simulink model "PV_string_with_MPPT"  (Simulink 8.8)
settings: Solver=ode3  StartTime=0.0  StopTime=600  FixedStep=1e-2  MaxStep=1e-4  RelTol=1e-5  EnableMultiTasking=on
(part 1 of 2)
settings Model: Creator=amaki  LastModifiedBy=jarvela7
settings DataIOCC: LimitDataPoints=off  SaveOutput=off  SaveTime=off
settings OptimizationCC: BooleanDataType=off  ExpressionDepthLimit=2147483647
settings DebuggingCC: AlgebraicLoopMsg=none
settings ConfigComp: CovSFcnEnable=off

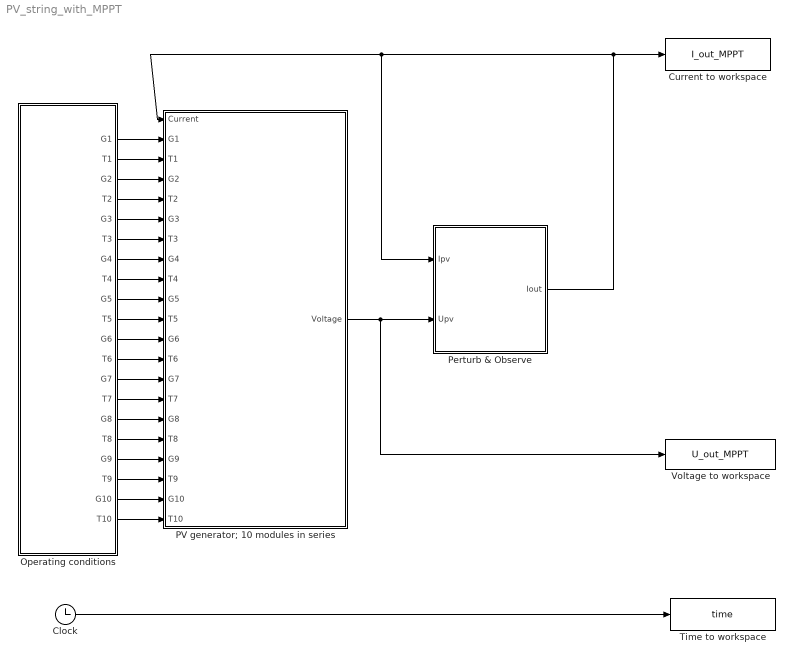
== system PV_string_with_MPPT ==
  Clock : Clock
  Current to workspace : ToWorkspace  VariableName=I_out_MPPT  SampleTime=-1
  Operating conditions : Subsystem
  PV generator; 10 modules in series : Subsystem
  Perturb & Observe : Subsystem  mask{pert_freq=1, pert_size=0.05}
      mask prompts: pert_freq "Perturbation frequency (Hz)"; pert_size "Perturbation step size (A)"
  Time to workspace : ToWorkspace  VariableName=time  SampleTime=-1
  Voltage to workspace : ToWorkspace  VariableName=U_out_MPPT  SampleTime=-1
  wires:
  Operating conditions/1(G1) -> PV generator; 10 modules in series/2(G1)
  Operating conditions/2(T1) -> PV generator; 10 modules in series/3(T1)
  Operating conditions/3(G2) -> PV generator; 10 modules in series/4(G2)
  Operating conditions/4(T2) -> PV generator; 10 modules in series/5(T2)
  Operating conditions/5(G3) -> PV generator; 10 modules in series/6(G3)
  Operating conditions/6(T3) -> PV generator; 10 modules in series/7(T3)
  Operating conditions/7(G4) -> PV generator; 10 modules in series/8(G4)
  Operating conditions/8(T4) -> PV generator; 10 modules in series/9(T4)
  Operating conditions/9(G5) -> PV generator; 10 modules in series/10(G5)
  Operating conditions/10(T5) -> PV generator; 10 modules in series/11(T5)
  Operating conditions/11(G6) -> PV generator; 10 modules in series/12(G6)
  Operating conditions/12(T6) -> PV generator; 10 modules in series/13(T6)
  Operating conditions/13(G7) -> PV generator; 10 modules in series/14(G7)
  Operating conditions/14(T7) -> PV generator; 10 modules in series/15(T7)
  Operating conditions/15(G8) -> PV generator; 10 modules in series/16(G8)
  Operating conditions/16(T8) -> PV generator; 10 modules in series/17(T8)
  Operating conditions/17(G9) -> PV generator; 10 modules in series/18(G9)
  Operating conditions/18(T9) -> PV generator; 10 modules in series/19(T9)
  Operating conditions/19(G10) -> PV generator; 10 modules in series/20(G10)
  Operating conditions/20(T10) -> PV generator; 10 modules in series/21(T10)
  Clock/1 -> Time to workspace/1
  PV generator; 10 modules in series/1(Voltage) -> Voltage to workspace/1, Perturb & Observe/2(Upv)
  Perturb & Observe/1(Iout) -> Current to workspace/1, PV generator; 10 modules in series/1(Current), Perturb & Observe/1(Ipv)

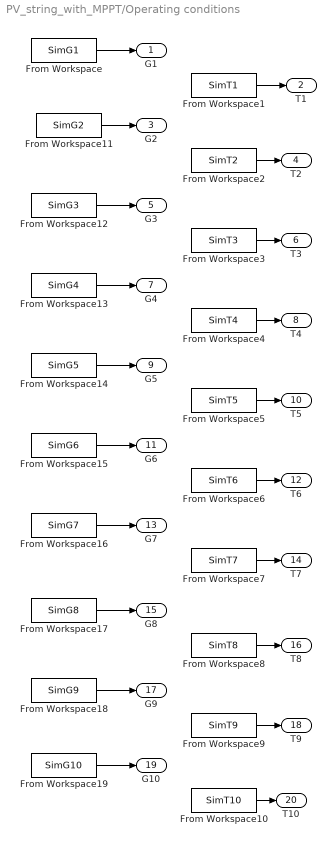
== system PV_string_with_MPPT/Operating conditions ==
  From Workspace : FromWorkspace  VariableName=SimG1  SampleTime=0
  From Workspace1 : FromWorkspace  VariableName=SimT1  SampleTime=0
  From Workspace10 : FromWorkspace  VariableName=SimT10  SampleTime=0
  From Workspace11 : FromWorkspace  VariableName=SimG2  SampleTime=0
  From Workspace12 : FromWorkspace  VariableName=SimG3  SampleTime=0
  From Workspace13 : FromWorkspace  VariableName=SimG4  SampleTime=0
  From Workspace14 : FromWorkspace  VariableName=SimG5  SampleTime=0
  From Workspace15 : FromWorkspace  VariableName=SimG6  SampleTime=0
  From Workspace16 : FromWorkspace  VariableName=SimG7  SampleTime=0
  From Workspace17 : FromWorkspace  VariableName=SimG8  SampleTime=0
  From Workspace18 : FromWorkspace  VariableName=SimG9  SampleTime=0
  From Workspace19 : FromWorkspace  VariableName=SimG10  SampleTime=0
  From Workspace2 : FromWorkspace  VariableName=SimT2  SampleTime=0
  From Workspace3 : FromWorkspace  VariableName=SimT3  SampleTime=0
  From Workspace4 : FromWorkspace  VariableName=SimT4  SampleTime=0
  From Workspace5 : FromWorkspace  VariableName=SimT5  SampleTime=0
  From Workspace6 : FromWorkspace  VariableName=SimT6  SampleTime=0
  From Workspace7 : FromWorkspace  VariableName=SimT7  SampleTime=0
  From Workspace8 : FromWorkspace  VariableName=SimT8  SampleTime=0
  From Workspace9 : FromWorkspace  VariableName=SimT9  SampleTime=0
  G1 : Outport
  T1 : Outport  Port=2
  G2 : Outport  Port=3
  T2 : Outport  Port=4
  G3 : Outport  Port=5
  T3 : Outport  Port=6
  G4 : Outport  Port=7
  T4 : Outport  Port=8
  G5 : Outport  Port=9
  T5 : Outport  Port=10
  G6 : Outport  Port=11
  T6 : Outport  Port=12
  G7 : Outport  Port=13
  T7 : Outport  Port=14
  G8 : Outport  Port=15
  T8 : Outport  Port=16
  G9 : Outport  Port=17
  T9 : Outport  Port=18
  G10 : Outport  Port=19
  T10 : Outport  Port=20
  wires:
  From Workspace1/1 -> T1/1
  From Workspace2/1 -> T2/1
  From Workspace3/1 -> T3/1
  From Workspace4/1 -> T4/1
  From Workspace5/1 -> T5/1
  From Workspace15/1 -> G6/1
  From Workspace6/1 -> T6/1
  From Workspace16/1 -> G7/1
  From Workspace7/1 -> T7/1
  From Workspace17/1 -> G8/1
  From Workspace8/1 -> T8/1
  From Workspace18/1 -> G9/1
  From Workspace9/1 -> T9/1
  From Workspace10/1 -> T10/1
  From Workspace19/1 -> G10/1
  From Workspace/1 -> G1/1
  From Workspace11/1 -> G2/1
  From Workspace12/1 -> G3/1
  From Workspace13/1 -> G4/1
  From Workspace14/1 -> G5/1

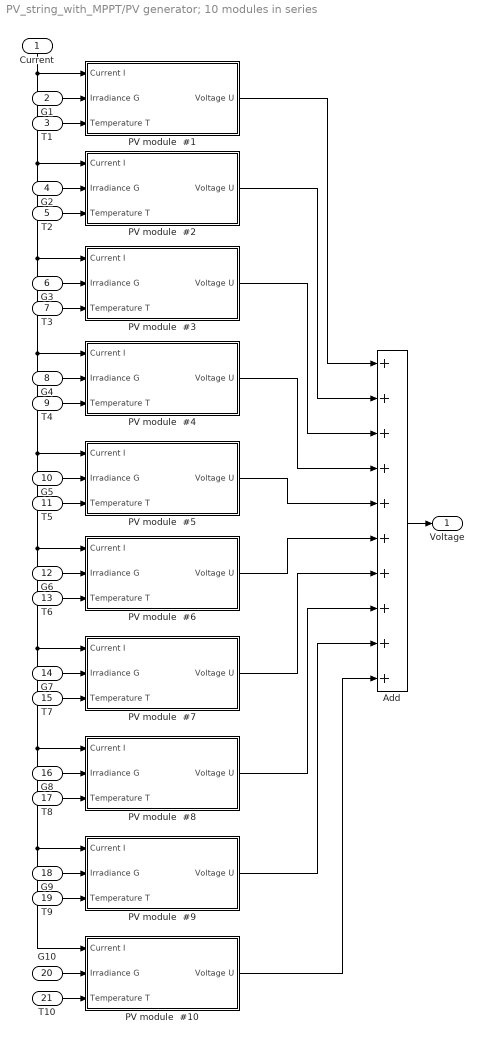
== system PV_string_with_MPPT/PV generator; 10 modules in series ==
  Current : Inport
  G1 : Inport  Port=2
  T1 : Inport  Port=3
  G2 : Inport  Port=4
  T2 : Inport  Port=5
  G3 : Inport  Port=6
  T3 : Inport  Port=7
  G4 : Inport  Port=8
  T4 : Inport  Port=9
  G5 : Inport  Port=10
  T5 : Inport  Port=11
  G6 : Inport  Port=12
  T6 : Inport  Port=13
  G7 : Inport  Port=14
  T7 : Inport  Port=15
  G8 : Inport  Port=16
  T8 : Inport  Port=17
  G9 : Inport  Port=18
  T9 : Inport  Port=19
  G10 : Inport  Port=20
  T10 : Inport  Port=21
  Add : Sum  Inputs=++++++++++
  PV module  #1 : Subsystem  mask{Isc_stc=8.02, Uoc_stc=33.1, G_stc=1000, T_stc=273.15+25, Ns=54, Rs=0.329385084266289, Rsh=187.8287416854189, A=1.3, Ku=-0.1242, Ki=0.0047, k=1.3806503e-23, q=1.60217646e-19}
      mask prompts: Isc_stc "STC short-circuit current"; Uoc_stc "STC open-circuit voltage"; G_stc "STC irradiance"; T_stc "STC temperature"; Ns "Number of cells"; Rs "Series resistance Rs"; Rsh "Shunt resistance Rsh"; A "Ideality factor A"; Ku "Temp. coeff. of OC Ku"; Ki "Temp. coeff. of SC Ki"; k "Boltzmann constant"; q "Elementary charge"
  PV module  #10 : Subsystem  mask{Isc_stc=8.02, Uoc_stc=33.1, G_stc=1000, T_stc=273.15+25, Ns=54, Rs=0.329385084266289, Rsh=187.8287416854189, A=1.3, Ku=-0.1242, Ki=0.0047, k=1.3806503e-23, q=1.60217646e-19}
      mask prompts: Isc_stc "STC short-circuit current"; Uoc_stc "STC open-circuit voltage"; G_stc "STC irradiance"; T_stc "STC temperature"; Ns "Number of cells"; Rs "Series resistance Rs"; Rsh "Shunt resistance Rsh"; A "Ideality factor A"; Ku "Temp. coeff. of OC Ku"; Ki "Temp. coeff. of SC Ki"; k "Boltzmann constant"; q "Elementary charge"
  PV module  #2 : Subsystem  mask{Isc_stc=8.02, Uoc_stc=33.1, G_stc=1000, T_stc=273.15+25, Ns=54, Rs=0.329385084266289, Rsh=187.8287416854189, A=1.3, Ku=-0.1242, Ki=0.0047, k=1.3806503e-23, q=1.60217646e-19}
      mask prompts: Isc_stc "STC short-circuit current"; Uoc_stc "STC open-circuit voltage"; G_stc "STC irradiance"; T_stc "STC temperature"; Ns "Number of cells"; Rs "Series resistance Rs"; Rsh "Shunt resistance Rsh"; A "Ideality factor A"; Ku "Temp. coeff. of OC Ku"; Ki "Temp. coeff. of SC Ki"; k "Boltzmann constant"; q "Elementary charge"
  PV module  #3 : Subsystem  mask{Isc_stc=8.02, Uoc_stc=33.1, G_stc=1000, T_stc=273.15+25, Ns=54, Rs=0.329385084266289, Rsh=187.8287416854189, A=1.3, Ku=-0.1242, Ki=0.0047, k=1.3806503e-23, q=1.60217646e-19}
      mask prompts: Isc_stc "STC short-circuit current"; Uoc_stc "STC open-circuit voltage"; G_stc "STC irradiance"; T_stc "STC temperature"; Ns "Number of cells"; Rs "Series resistance Rs"; Rsh "Shunt resistance Rsh"; A "Ideality factor A"; Ku "Temp. coeff. of OC Ku"; Ki "Temp. coeff. of SC Ki"; k "Boltzmann constant"; q "Elementary charge"
  PV module  #4 : Subsystem  mask{Isc_stc=8.02, Uoc_stc=33.1, G_stc=1000, T_stc=273.15+25, Ns=54, Rs=0.329385084266289, Rsh=187.8287416854189, A=1.3, Ku=-0.1242, Ki=0.0047, k=1.3806503e-23, q=1.60217646e-19}
      mask prompts: Isc_stc "STC short-circuit current"; Uoc_stc "STC open-circuit voltage"; G_stc "STC irradiance"; T_stc "STC temperature"; Ns "Number of cells"; Rs "Series resistance Rs"; Rsh "Shunt resistance Rsh"; A "Ideality factor A"; Ku "Temp. coeff. of OC Ku"; Ki "Temp. coeff. of SC Ki"; k "Boltzmann constant"; q "Elementary charge"
  PV module  #5 : Subsystem  mask{Isc_stc=8.02, Uoc_stc=33.1, G_stc=1000, T_stc=273.15+25, Ns=54, Rs=0.329385084266289, Rsh=187.8287416854189, A=1.3, Ku=-0.1242, Ki=0.0047, k=1.3806503e-23, q=1.60217646e-19}
      mask prompts: Isc_stc "STC short-circuit current"; Uoc_stc "STC open-circuit voltage"; G_stc "STC irradiance"; T_stc "STC temperature"; Ns "Number of cells"; Rs "Series resistance Rs"; Rsh "Shunt resistance Rsh"; A "Ideality factor A"; Ku "Temp. coeff. of OC Ku"; Ki "Temp. coeff. of SC Ki"; k "Boltzmann constant"; q "Elementary charge"
  PV module  #6 : Subsystem  mask{Isc_stc=8.02, Uoc_stc=33.1, G_stc=1000, T_stc=273.15+25, Ns=54, Rs=0.329385084266289, Rsh=187.8287416854189, A=1.3, Ku=-0.1242, Ki=0.0047, k=1.3806503e-23, q=1.60217646e-19}
      mask prompts: Isc_stc "STC short-circuit current"; Uoc_stc "STC open-circuit voltage"; G_stc "STC irradiance"; T_stc "STC temperature"; Ns "Number of cells"; Rs "Series resistance Rs"; Rsh "Shunt resistance Rsh"; A "Ideality factor A"; Ku "Temp. coeff. of OC Ku"; Ki "Temp. coeff. of SC Ki"; k "Boltzmann constant"; q "Elementary charge"
  PV module  #7 : Subsystem  mask{Isc_stc=8.02, Uoc_stc=33.1, G_stc=1000, T_stc=273.15+25, Ns=54, Rs=0.329385084266289, Rsh=187.8287416854189, A=1.3, Ku=-0.1242, Ki=0.0047, k=1.3806503e-23, q=1.60217646e-19}
      mask prompts: Isc_stc "STC short-circuit current"; Uoc_stc "STC open-circuit voltage"; G_stc "STC irradiance"; T_stc "STC temperature"; Ns "Number of cells"; Rs "Series resistance Rs"; Rsh "Shunt resistance Rsh"; A "Ideality factor A"; Ku "Temp. coeff. of OC Ku"; Ki "Temp. coeff. of SC Ki"; k "Boltzmann constant"; q "Elementary charge"
  PV module  #8 : Subsystem  mask{Isc_stc=8.02, Uoc_stc=33.1, G_stc=1000, T_stc=273.15+25, Ns=54, Rs=0.329385084266289, Rsh=187.8287416854189, A=1.3, Ku=-0.1242, Ki=0.0047, k=1.3806503e-23, q=1.60217646e-19}
      mask prompts: Isc_stc "STC short-circuit current"; Uoc_stc "STC open-circuit voltage"; G_stc "STC irradiance"; T_stc "STC temperature"; Ns "Number of cells"; Rs "Series resistance Rs"; Rsh "Shunt resistance Rsh"; A "Ideality factor A"; Ku "Temp. coeff. of OC Ku"; Ki "Temp. coeff. of SC Ki"; k "Boltzmann constant"; q "Elementary charge"
  PV module  #9 : Subsystem  mask{Isc_stc=8.02, Uoc_stc=33.1, G_stc=1000, T_stc=273.15+25, Ns=54, Rs=0.329385084266289, Rsh=187.8287416854189, A=1.3, Ku=-0.1242, Ki=0.0047, k=1.3806503e-23, q=1.60217646e-19}
      mask prompts: Isc_stc "STC short-circuit current"; Uoc_stc "STC open-circuit voltage"; G_stc "STC irradiance"; T_stc "STC temperature"; Ns "Number of cells"; Rs "Series resistance Rs"; Rsh "Shunt resistance Rsh"; A "Ideality factor A"; Ku "Temp. coeff. of OC Ku"; Ki "Temp. coeff. of SC Ki"; k "Boltzmann constant"; q "Elementary charge"
  Voltage : Outport
  wires:
  PV module  #1/1(Voltage U) -> Add/1
  PV module  #2/1(Voltage U) -> Add/2
  PV module  #3/1(Voltage U) -> Add/3
  PV module  #4/1(Voltage U) -> Add/4
  PV module  #5/1(Voltage U) -> Add/5
  PV module  #6/1(Voltage U) -> Add/6
  PV module  #7/1(Voltage U) -> Add/7
  PV module  #8/1(Voltage U) -> Add/8
  PV module  #9/1(Voltage U) -> Add/9
  PV module  #10/1(Voltage U) -> Add/10
  Current/1 -> PV module  #1/1(Current I), PV module  #2/1(Current I), PV module  #3/1(Current I), PV module  #4/1(Current I), PV module  #5/1(Current I), PV module  #6/1(Current I), PV module  #7/1(Current I), PV module  #8/1(Current I), PV module  #9/1(Current I), PV module  #10/1(Current I)
  G1/1 -> PV module  #1/2(Irradiance G)
  T1/1 -> PV module  #1/3(Temperature T)
  G2/1 -> PV module  #2/2(Irradiance G)
  T2/1 -> PV module  #2/3(Temperature T)
  G3/1 -> PV module  #3/2(Irradiance G)
  T3/1 -> PV module  #3/3(Temperature T)
  G4/1 -> PV module  #4/2(Irradiance G)
  T4/1 -> PV module  #4/3(Temperature T)
  G5/1 -> PV module  #5/2(Irradiance G)
  T5/1 -> PV module  #5/3(Temperature T)
  Add/1 -> Voltage/1
  G6/1 -> PV module  #6/2(Irradiance G)
  T6/1 -> PV module  #6/3(Temperature T)
  G7/1 -> PV module  #7/2(Irradiance G)
  T7/1 -> PV module  #7/3(Temperature T)
  G8/1 -> PV module  #8/2(Irradiance G)
  T8/1 -> PV module  #8/3(Temperature T)
  G9/1 -> PV module  #9/2(Irradiance G)
  T9/1 -> PV module  #9/3(Temperature T)
  G10/1 -> PV module  #10/2(Irradiance G)
  T10/1 -> PV module  #10/3(Temperature T)

== system PV_string_with_MPPT/Perturb & Observe ==
  Ipv : Inport
  Upv : Inport  Port=2
  Memory : Memory  InheritSampleTime=on
  Memory1 : Memory  InheritSampleTime=on
  Memory3 : Memory  X0=0.1  InheritSampleTime=on
  P : Product  RndMeth=Zero
  Product : Product  RndMeth=Zero
  Product1 : Product  RndMeth=Zero
  Rate Transition : RateTransition  OutPortSampleTime=1e-2
  Saturation : Saturate  UpperLimit=inf  LowerLimit=0
  Sign : Signum
  Sign1 : Signum
  Sign2 : Signum
  Sum : Sum  Inputs=|++
  Zero-Order Hold : ZeroOrderHold  SampleTime=1/pert_freq
  Zero-Order Hold1 : ZeroOrderHold  SampleTime=1/pert_freq
  dp : Sum  Inputs=+-
  du : Sum  Inputs=+-
  step : Constant  Value=-pert_size
  Iout : Outport
  wires:
  Memory1/1 -> du/2
  Memory/1 -> dp/2
  Upv/1 -> Zero-Order Hold1/1
  du/1 -> Sign1/1
  step/1 -> Product/2
  Product/1 -> Sum/1
  Sign/1 -> Product1/1
  Sign1/1 -> Product1/2
  Product1/1 -> Sign2/1
  Ipv/1 -> Zero-Order Hold/1
  Zero-Order Hold1/1 -> P/2, Memory1/1, du/1
  Zero-Order Hold/1 -> P/1
  P/1 -> Memory/1, dp/1
  dp/1 -> Sign/1
  Sign2/1 -> Product/1
  Sum/1 -> Rate Transition/1, Memory3/1
  Rate Transition/1 -> Saturation/1
  Memory3/1 -> Sum/2
  Saturation/1 -> Iout/1

== system PV_string_with_MPPT/PV generator; 10 modules in series/PV module  #1 ==
  Current I : Inport
  Irradiance G : Inport  Port=2
  Temperature T : Inport  Port=3
  Add1 : Sum  Inputs=-+
  Bypass diode : Subsystem  mask{k=1.3806503e-23, q=1.60217646e-19, Rs_bypass=0.02}
      mask prompts: k "Boltzmann constant"; q "Elementary charge"; Rs_bypass "Series resistance"
  MinMax : MinMax  Function=max  Inputs=2
  Pv module : Subsystem
  Voltage U : Outport
  wires:
  MinMax/1 -> Voltage U/1
  Add1/1 -> Bypass diode/1(I)
  Bypass diode/1(Ubypass) -> MinMax/2
  Pv module/2(Isc) -> Add1/1
  Pv module/1(U) -> MinMax/1
  Irradiance G/1 -> Pv module/1(G)
  Temperature T/1 -> Pv module/2(T)
  Current I/1 -> Pv module/3(I), Add1/2

== system PV_string_with_MPPT/PV generator; 10 modules in series/PV module  #10 ==
  Current I : Inport
  Irradiance G : Inport  Port=2
  Temperature T : Inport  Port=3
  Add1 : Sum  Inputs=-+
  Bypass diode : Subsystem  mask{k=1.3806503e-23, q=1.60217646e-19, Rs_bypass=0.02}
      mask prompts: k "Boltzmann constant"; q "Elementary charge"; Rs_bypass "Series resistance"
  MinMax : MinMax  Function=max  Inputs=2
  Pv module : Subsystem
  Voltage U : Outport
  wires:
  MinMax/1 -> Voltage U/1
  Add1/1 -> Bypass diode/1(I)
  Bypass diode/1(Ubypass) -> MinMax/2
  Pv module/2(Isc) -> Add1/1
  Pv module/1(U) -> MinMax/1
  Irradiance G/1 -> Pv module/1(G)
  Temperature T/1 -> Pv module/2(T)
  Current I/1 -> Pv module/3(I), Add1/2

== system PV_string_with_MPPT/PV generator; 10 modules in series/PV module  #2 ==
  Current I : Inport
  Irradiance G : Inport  Port=2
  Temperature T : Inport  Port=3
  Add1 : Sum  Inputs=-+
  Bypass diode : Subsystem  mask{k=1.3806503e-23, q=1.60217646e-19, Rs_bypass=0.02}
      mask prompts: k "Boltzmann constant"; q "Elementary charge"; Rs_bypass "Series resistance"
  MinMax : MinMax  Function=max  Inputs=2
  Pv module : Subsystem
  Voltage U : Outport
  wires:
  Current I/1 -> Add1/2, Pv module/3(I)
  Temperature T/1 -> Pv module/2(T)
  Irradiance G/1 -> Pv module/1(G)
  Pv module/1(U) -> MinMax/1
  Pv module/2(Isc) -> Add1/1
  Bypass diode/1(Ubypass) -> MinMax/2
  Add1/1 -> Bypass diode/1(I)
  MinMax/1 -> Voltage U/1

== system PV_string_with_MPPT/PV generator; 10 modules in series/PV module  #3 ==
  Current I : Inport
  Irradiance G : Inport  Port=2
  Temperature T : Inport  Port=3
  Add1 : Sum  Inputs=-+
  Bypass diode : Subsystem  mask{k=1.3806503e-23, q=1.60217646e-19, Rs_bypass=0.02}
      mask prompts: k "Boltzmann constant"; q "Elementary charge"; Rs_bypass "Series resistance"
  MinMax : MinMax  Function=max  Inputs=2
  Pv module : Subsystem
  Voltage U : Outport
  wires:
  MinMax/1 -> Voltage U/1
  Add1/1 -> Bypass diode/1(I)
  Bypass diode/1(Ubypass) -> MinMax/2
  Pv module/2(Isc) -> Add1/1
  Pv module/1(U) -> MinMax/1
  Irradiance G/1 -> Pv module/1(G)
  Temperature T/1 -> Pv module/2(T)
  Current I/1 -> Pv module/3(I), Add1/2

== system PV_string_with_MPPT/PV generator; 10 modules in series/PV module  #4 ==
  Current I : Inport
  Irradiance G : Inport  Port=2
  Temperature T : Inport  Port=3
  Add1 : Sum  Inputs=-+
  Bypass diode : Subsystem  mask{k=1.3806503e-23, q=1.60217646e-19, Rs_bypass=0.02}
      mask prompts: k "Boltzmann constant"; q "Elementary charge"; Rs_bypass "Series resistance"
  MinMax : MinMax  Function=max  Inputs=2
  Pv module : Subsystem
  Voltage U : Outport
  wires:
  Current I/1 -> Add1/2, Pv module/3(I)
  Temperature T/1 -> Pv module/2(T)
  Irradiance G/1 -> Pv module/1(G)
  Pv module/1(U) -> MinMax/1
  Pv module/2(Isc) -> Add1/1
  Bypass diode/1(Ubypass) -> MinMax/2
  Add1/1 -> Bypass diode/1(I)
  MinMax/1 -> Voltage U/1

== system PV_string_with_MPPT/PV generator; 10 modules in series/PV module  #5 ==
  Current I : Inport
  Irradiance G : Inport  Port=2
  Temperature T : Inport  Port=3
  Add1 : Sum  Inputs=-+
  Bypass diode : Subsystem  mask{k=1.3806503e-23, q=1.60217646e-19, Rs_bypass=0.02}
      mask prompts: k "Boltzmann constant"; q "Elementary charge"; Rs_bypass "Series resistance"
  MinMax : MinMax  Function=max  Inputs=2
  Pv module : Subsystem
  Voltage U : Outport
  wires:
  MinMax/1 -> Voltage U/1
  Add1/1 -> Bypass diode/1(I)
  Bypass diode/1(Ubypass) -> MinMax/2
  Pv module/2(Isc) -> Add1/1
  Pv module/1(U) -> MinMax/1
  Irradiance G/1 -> Pv module/1(G)
  Temperature T/1 -> Pv module/2(T)
  Current I/1 -> Pv module/3(I), Add1/2

== system PV_string_with_MPPT/PV generator; 10 modules in series/PV module  #6 ==
  Current I : Inport
  Irradiance G : Inport  Port=2
  Temperature T : Inport  Port=3
  Add1 : Sum  Inputs=-+
  Bypass diode : Subsystem  mask{k=1.3806503e-23, q=1.60217646e-19, Rs_bypass=0.02}
      mask prompts: k "Boltzmann constant"; q "Elementary charge"; Rs_bypass "Series resistance"
  MinMax : MinMax  Function=max  Inputs=2
  Pv module : Subsystem
  Voltage U : Outport
  wires:
  Current I/1 -> Add1/2, Pv module/3(I)
  Temperature T/1 -> Pv module/2(T)
  Irradiance G/1 -> Pv module/1(G)
  Pv module/1(U) -> MinMax/1
  Pv module/2(Isc) -> Add1/1
  Bypass diode/1(Ubypass) -> MinMax/2
  Add1/1 -> Bypass diode/1(I)
  MinMax/1 -> Voltage U/1

== system PV_string_with_MPPT/PV generator; 10 modules in series/PV module  #7 ==
  Current I : Inport
  Irradiance G : Inport  Port=2
  Temperature T : Inport  Port=3
  Add1 : Sum  Inputs=-+
  Bypass diode : Subsystem  mask{k=1.3806503e-23, q=1.60217646e-19, Rs_bypass=0.02}
      mask prompts: k "Boltzmann constant"; q "Elementary charge"; Rs_bypass "Series resistance"
  MinMax : MinMax  Function=max  Inputs=2
  Pv module : Subsystem
  Voltage U : Outport
  wires:
  Current I/1 -> Add1/2, Pv module/3(I)
  Temperature T/1 -> Pv module/2(T)
  Irradiance G/1 -> Pv module/1(G)
  Pv module/1(U) -> MinMax/1
  Pv module/2(Isc) -> Add1/1
  Bypass diode/1(Ubypass) -> MinMax/2
  Add1/1 -> Bypass diode/1(I)
  MinMax/1 -> Voltage U/1

== system PV_string_with_MPPT/PV generator; 10 modules in series/PV module  #8 ==
  Current I : Inport
  Irradiance G : Inport  Port=2
  Temperature T : Inport  Port=3
  Add1 : Sum  Inputs=-+
  Bypass diode : Subsystem  mask{k=1.3806503e-23, q=1.60217646e-19, Rs_bypass=0.02}
      mask prompts: k "Boltzmann constant"; q "Elementary charge"; Rs_bypass "Series resistance"
  MinMax : MinMax  Function=max  Inputs=2
  Pv module : Subsystem
  Voltage U : Outport
  wires:
  MinMax/1 -> Voltage U/1
  Add1/1 -> Bypass diode/1(I)
  Bypass diode/1(Ubypass) -> MinMax/2
  Pv module/2(Isc) -> Add1/1
  Pv module/1(U) -> MinMax/1
  Irradiance G/1 -> Pv module/1(G)
  Temperature T/1 -> Pv module/2(T)
  Current I/1 -> Pv module/3(I), Add1/2

== system PV_string_with_MPPT/PV generator; 10 modules in series/PV module  #9 ==
  Current I : Inport
  Irradiance G : Inport  Port=2
  Temperature T : Inport  Port=3
  Add1 : Sum  Inputs=-+
  Bypass diode : Subsystem  mask{k=1.3806503e-23, q=1.60217646e-19, Rs_bypass=0.02}
      mask prompts: k "Boltzmann constant"; q "Elementary charge"; Rs_bypass "Series resistance"
  MinMax : MinMax  Function=max  Inputs=2
  Pv module : Subsystem
  Voltage U : Outport
  wires:
  Current I/1 -> Add1/2, Pv module/3(I)
  Temperature T/1 -> Pv module/2(T)
  Irradiance G/1 -> Pv module/1(G)
  Pv module/1(U) -> MinMax/1
  Pv module/2(Isc) -> Add1/1
  Bypass diode/1(Ubypass) -> MinMax/2
  Add1/1 -> Bypass diode/1(I)
  MinMax/1 -> Voltage U/1

== system PV_string_with_MPPT/PV generator; 10 modules in series/PV module  #1/Bypass diode ==
  I : Inport
  Bypass diode junction temperature : Constant  Value=298
  Bypass diode saturation current : Constant  Value=3.2e-6
  Divide4 : Product  Inputs=/*
  Gain1 : Gain  Gain=Rs_bypass
  Gain2 : Gain  Gain=-1
  Gain9 : Gain  Gain=1.5
  Math Function2 : Math  Operator=log  SaturateOnIntegerOverflow=on
  Product2 : Product  RndMeth=Zero
  Saturation1 : Saturate  UpperLimit=1e24  LowerLimit=0
  Subtract : Sum
  Subtract5 : Sum
  Thermal voltage : Subsystem
  Ubypass : Outport
  wires:
  Gain2/1 -> Ubypass/1
  Subtract/1 -> Gain2/1
  Saturation1/1 -> Gain1/1, Subtract5/2
  Subtract5/1 -> Divide4/2
  Divide4/1 -> Math Function2/1
  Bypass diode junction temperature/1 -> Thermal voltage/1(T)
  Gain1/1 -> Subtract/2
  Product2/1 -> Subtract/1
  I/1 -> Saturation1/1
  Bypass diode saturation current/1 -> Divide4/1, Subtract5/1
  Thermal voltage/1(Vt) -> Gain9/1
  Gain9/1 -> Product2/1
  Math Function2/1 -> Product2/2

== system PV_string_with_MPPT/PV generator; 10 modules in series/PV module  #1/Pv module ==
  G : Inport
  T : Inport  Port=2
  I : Inport  Port=3
  Add1 : Sum  Inputs=+--
  Gain1 : Gain  Gain=Rsh
  Gain3 : Gain  Gain=(Rsh+Rs)/Rsh
  Subsystem : Subsystem
  Subsystem1 : Subsystem
  U : Outport
  Isc : Outport  Port=2
  wires:
  Subsystem/1(Isc) -> Isc/1
  Gain1/1 -> U/1, Subsystem1/2(U)
  Add1/1 -> Gain1/1
  Gain3/1 -> Add1/3
  I/1 -> Gain3/1, Subsystem1/3(I)
  Subsystem1/1(Id) -> Add1/2
  T/1 -> Subsystem1/1(T), Subsystem/2(T)
  G/1 -> Subsystem/1(G)
  Subsystem/2(Ipv) -> Add1/1

== system PV_string_with_MPPT/PV generator; 10 modules in series/PV module  #10/Bypass diode ==
  I : Inport
  Bypass diode junction temperature : Constant  Value=298
  Bypass diode saturation current : Constant  Value=3.2e-6
  Divide4 : Product  Inputs=/*
  Gain1 : Gain  Gain=Rs_bypass
  Gain2 : Gain  Gain=-1
  Gain9 : Gain  Gain=1.5
  Math Function2 : Math  Operator=log  SaturateOnIntegerOverflow=on
  Product2 : Product  RndMeth=Zero
  Saturation1 : Saturate  UpperLimit=1e24  LowerLimit=0
  Subtract : Sum
  Subtract5 : Sum
  Thermal voltage : Subsystem
  Ubypass : Outport
  wires:
  Gain2/1 -> Ubypass/1
  Subtract/1 -> Gain2/1
  Saturation1/1 -> Gain1/1, Subtract5/2
  Subtract5/1 -> Divide4/2
  Divide4/1 -> Math Function2/1
  Bypass diode junction temperature/1 -> Thermal voltage/1(T)
  Gain1/1 -> Subtract/2
  Product2/1 -> Subtract/1
  I/1 -> Saturation1/1
  Bypass diode saturation current/1 -> Divide4/1, Subtract5/1
  Thermal voltage/1(Vt) -> Gain9/1
  Gain9/1 -> Product2/1
  Math Function2/1 -> Product2/2

== system PV_string_with_MPPT/PV generator; 10 modules in series/PV module  #10/Pv module ==
  G : Inport
  T : Inport  Port=2
  I : Inport  Port=3
  Add1 : Sum  Inputs=+--
  Gain1 : Gain  Gain=Rsh
  Gain3 : Gain  Gain=(Rsh+Rs)/Rsh
  Subsystem : Subsystem
  Subsystem1 : Subsystem
  U : Outport
  Isc : Outport  Port=2
  wires:
  Subsystem/1(Isc) -> Isc/1
  Gain1/1 -> U/1, Subsystem1/2(U)
  Add1/1 -> Gain1/1
  Gain3/1 -> Add1/3
  I/1 -> Gain3/1, Subsystem1/3(I)
  Subsystem1/1(Id) -> Add1/2
  T/1 -> Subsystem1/1(T), Subsystem/2(T)
  G/1 -> Subsystem/1(G)
  Subsystem/2(Ipv) -> Add1/1

== system PV_string_with_MPPT/PV generator; 10 modules in series/PV module  #2/Bypass diode ==
  I : Inport
  Bypass diode junction temperature : Constant  Value=298
  Bypass diode saturation current : Constant  Value=3.2e-6
  Divide4 : Product  Inputs=/*
  Gain1 : Gain  Gain=Rs_bypass
  Gain2 : Gain  Gain=-1
  Gain9 : Gain  Gain=1.5
  Math Function2 : Math  Operator=log  SaturateOnIntegerOverflow=on
  Product2 : Product  RndMeth=Zero
  Saturation1 : Saturate  UpperLimit=1e24  LowerLimit=0
  Subtract : Sum
  Subtract5 : Sum
  Thermal voltage : Subsystem
  Ubypass : Outport
  wires:
  Math Function2/1 -> Product2/2
  Gain9/1 -> Product2/1
  Thermal voltage/1(Vt) -> Gain9/1
  Bypass diode saturation current/1 -> Subtract5/1, Divide4/1
  I/1 -> Saturation1/1
  Product2/1 -> Subtract/1
  Gain1/1 -> Subtract/2
  Bypass diode junction temperature/1 -> Thermal voltage/1(T)
  Divide4/1 -> Math Function2/1
  Subtract5/1 -> Divide4/2
  Saturation1/1 -> Subtract5/2, Gain1/1
  Subtract/1 -> Gain2/1
  Gain2/1 -> Ubypass/1

== system PV_string_with_MPPT/PV generator; 10 modules in series/PV module  #2/Pv module ==
  G : Inport
  T : Inport  Port=2
  I : Inport  Port=3
  Add1 : Sum  Inputs=+--
  Gain1 : Gain  Gain=Rsh
  Gain3 : Gain  Gain=(Rsh+Rs)/Rsh
  Subsystem : Subsystem
  Subsystem1 : Subsystem
  U : Outport
  Isc : Outport  Port=2
  wires:
  Subsystem/2(Ipv) -> Add1/1
  G/1 -> Subsystem/1(G)
  T/1 -> Subsystem/2(T), Subsystem1/1(T)
  Subsystem1/1(Id) -> Add1/2
  I/1 -> Subsystem1/3(I), Gain3/1
  Gain3/1 -> Add1/3
  Add1/1 -> Gain1/1
  Gain1/1 -> Subsystem1/2(U), U/1
  Subsystem/1(Isc) -> Isc/1

== system PV_string_with_MPPT/PV generator; 10 modules in series/PV module  #3/Bypass diode ==
  I : Inport
  Bypass diode junction temperature : Constant  Value=298
  Bypass diode saturation current : Constant  Value=3.2e-6
  Divide4 : Product  Inputs=/*
  Gain1 : Gain  Gain=Rs_bypass
  Gain2 : Gain  Gain=-1
  Gain9 : Gain  Gain=1.5
  Math Function2 : Math  Operator=log  SaturateOnIntegerOverflow=on
  Product2 : Product  RndMeth=Zero
  Saturation1 : Saturate  UpperLimit=1e24  LowerLimit=0
  Subtract : Sum
  Subtract5 : Sum
  Thermal voltage : Subsystem
  Ubypass : Outport
  wires:
  Gain2/1 -> Ubypass/1
  Subtract/1 -> Gain2/1
  Saturation1/1 -> Gain1/1, Subtract5/2
  Subtract5/1 -> Divide4/2
  Divide4/1 -> Math Function2/1
  Bypass diode junction temperature/1 -> Thermal voltage/1(T)
  Gain1/1 -> Subtract/2
  Product2/1 -> Subtract/1
  I/1 -> Saturation1/1
  Bypass diode saturation current/1 -> Divide4/1, Subtract5/1
  Thermal voltage/1(Vt) -> Gain9/1
  Gain9/1 -> Product2/1
  Math Function2/1 -> Product2/2

== system PV_string_with_MPPT/PV generator; 10 modules in series/PV module  #3/Pv module ==
  G : Inport
  T : Inport  Port=2
  I : Inport  Port=3
  Add1 : Sum  Inputs=+--
  Gain1 : Gain  Gain=Rsh
  Gain3 : Gain  Gain=(Rsh+Rs)/Rsh
  Subsystem : Subsystem
  Subsystem1 : Subsystem
  U : Outport
  Isc : Outport  Port=2
  wires:
  Subsystem/1(Isc) -> Isc/1
  Gain1/1 -> U/1, Subsystem1/2(U)
  Add1/1 -> Gain1/1
  Gain3/1 -> Add1/3
  I/1 -> Gain3/1, Subsystem1/3(I)
  Subsystem1/1(Id) -> Add1/2
  T/1 -> Subsystem1/1(T), Subsystem/2(T)
  G/1 -> Subsystem/1(G)
  Subsystem/2(Ipv) -> Add1/1

== system PV_string_with_MPPT/PV generator; 10 modules in series/PV module  #4/Bypass diode ==
  I : Inport
  Bypass diode junction temperature : Constant  Value=298
  Bypass diode saturation current : Constant  Value=3.2e-6
  Divide4 : Product  Inputs=/*
  Gain1 : Gain  Gain=Rs_bypass
  Gain2 : Gain  Gain=-1
  Gain9 : Gain  Gain=1.5
  Math Function2 : Math  Operator=log  SaturateOnIntegerOverflow=on
  Product2 : Product  RndMeth=Zero
  Saturation1 : Saturate  UpperLimit=1e24  LowerLimit=0
  Subtract : Sum
  Subtract5 : Sum
  Thermal voltage : Subsystem
  Ubypass : Outport
  wires:
  Math Function2/1 -> Product2/2
  Gain9/1 -> Product2/1
  Thermal voltage/1(Vt) -> Gain9/1
  Bypass diode saturation current/1 -> Subtract5/1, Divide4/1
  I/1 -> Saturation1/1
  Product2/1 -> Subtract/1
  Gain1/1 -> Subtract/2
  Bypass diode junction temperature/1 -> Thermal voltage/1(T)
  Divide4/1 -> Math Function2/1
  Subtract5/1 -> Divide4/2
  Saturation1/1 -> Subtract5/2, Gain1/1
  Subtract/1 -> Gain2/1
  Gain2/1 -> Ubypass/1

== system PV_string_with_MPPT/PV generator; 10 modules in series/PV module  #4/Pv module ==
  G : Inport
  T : Inport  Port=2
  I : Inport  Port=3
  Add1 : Sum  Inputs=+--
  Gain1 : Gain  Gain=Rsh
  Gain3 : Gain  Gain=(Rsh+Rs)/Rsh
  Subsystem : Subsystem
  Subsystem1 : Subsystem
  U : Outport
  Isc : Outport  Port=2
  wires:
  Subsystem/2(Ipv) -> Add1/1
  G/1 -> Subsystem/1(G)
  T/1 -> Subsystem/2(T), Subsystem1/1(T)
  Subsystem1/1(Id) -> Add1/2
  I/1 -> Subsystem1/3(I), Gain3/1
  Gain3/1 -> Add1/3
  Add1/1 -> Gain1/1
  Gain1/1 -> Subsystem1/2(U), U/1
  Subsystem/1(Isc) -> Isc/1

== system PV_string_with_MPPT/PV generator; 10 modules in series/PV module  #5/Bypass diode ==
  I : Inport
  Bypass diode junction temperature : Constant  Value=298
  Bypass diode saturation current : Constant  Value=3.2e-6
  Divide4 : Product  Inputs=/*
  Gain1 : Gain  Gain=Rs_bypass
  Gain2 : Gain  Gain=-1
  Gain9 : Gain  Gain=1.5
  Math Function2 : Math  Operator=log  SaturateOnIntegerOverflow=on
  Product2 : Product  RndMeth=Zero
  Saturation1 : Saturate  UpperLimit=1e24  LowerLimit=0
  Subtract : Sum
  Subtract5 : Sum
  Thermal voltage : Subsystem
  Ubypass : Outport
  wires:
  Gain2/1 -> Ubypass/1
  Subtract/1 -> Gain2/1
  Saturation1/1 -> Gain1/1, Subtract5/2
  Subtract5/1 -> Divide4/2
  Divide4/1 -> Math Function2/1
  Bypass diode junction temperature/1 -> Thermal voltage/1(T)
  Gain1/1 -> Subtract/2
  Product2/1 -> Subtract/1
  I/1 -> Saturation1/1
  Bypass diode saturation current/1 -> Divide4/1, Subtract5/1
  Thermal voltage/1(Vt) -> Gain9/1
  Gain9/1 -> Product2/1
  Math Function2/1 -> Product2/2

== system PV_string_with_MPPT/PV generator; 10 modules in series/PV module  #5/Pv module ==
  G : Inport
  T : Inport  Port=2
  I : Inport  Port=3
  Add1 : Sum  Inputs=+--
  Gain1 : Gain  Gain=Rsh
  Gain3 : Gain  Gain=(Rsh+Rs)/Rsh
  Subsystem : Subsystem
  Subsystem1 : Subsystem
  U : Outport
  Isc : Outport  Port=2
  wires:
  Subsystem/1(Isc) -> Isc/1
  Gain1/1 -> U/1, Subsystem1/2(U)
  Add1/1 -> Gain1/1
  Gain3/1 -> Add1/3
  I/1 -> Gain3/1, Subsystem1/3(I)
  Subsystem1/1(Id) -> Add1/2
  T/1 -> Subsystem1/1(T), Subsystem/2(T)
  G/1 -> Subsystem/1(G)
  Subsystem/2(Ipv) -> Add1/1

== system PV_string_with_MPPT/PV generator; 10 modules in series/PV module  #6/Bypass diode ==
  I : Inport
  Bypass diode junction temperature : Constant  Value=298
  Bypass diode saturation current : Constant  Value=3.2e-6
  Divide4 : Product  Inputs=/*
  Gain1 : Gain  Gain=Rs_bypass
  Gain2 : Gain  Gain=-1
  Gain9 : Gain  Gain=1.5
  Math Function2 : Math  Operator=log  SaturateOnIntegerOverflow=on
  Product2 : Product  RndMeth=Zero
  Saturation1 : Saturate  UpperLimit=1e24  LowerLimit=0
  Subtract : Sum
  Subtract5 : Sum
  Thermal voltage : Subsystem
  Ubypass : Outport
  wires:
  Math Function2/1 -> Product2/2
  Gain9/1 -> Product2/1
  Thermal voltage/1(Vt) -> Gain9/1
  Bypass diode saturation current/1 -> Subtract5/1, Divide4/1
  I/1 -> Saturation1/1
  Product2/1 -> Subtract/1
  Gain1/1 -> Subtract/2
  Bypass diode junction temperature/1 -> Thermal voltage/1(T)
  Divide4/1 -> Math Function2/1
  Subtract5/1 -> Divide4/2
  Saturation1/1 -> Subtract5/2, Gain1/1
  Subtract/1 -> Gain2/1
  Gain2/1 -> Ubypass/1

== system PV_string_with_MPPT/PV generator; 10 modules in series/PV module  #6/Pv module ==
  G : Inport
  T : Inport  Port=2
  I : Inport  Port=3
  Add1 : Sum  Inputs=+--
  Gain1 : Gain  Gain=Rsh
  Gain3 : Gain  Gain=(Rsh+Rs)/Rsh
  Subsystem : Subsystem
  Subsystem1 : Subsystem
  U : Outport
  Isc : Outport  Port=2
  wires:
  Subsystem/2(Ipv) -> Add1/1
  G/1 -> Subsystem/1(G)
  T/1 -> Subsystem/2(T), Subsystem1/1(T)
  Subsystem1/1(Id) -> Add1/2
  I/1 -> Subsystem1/3(I), Gain3/1
  Gain3/1 -> Add1/3
  Add1/1 -> Gain1/1
  Gain1/1 -> Subsystem1/2(U), U/1
  Subsystem/1(Isc) -> Isc/1

== system PV_string_with_MPPT/PV generator; 10 modules in series/PV module  #7/Bypass diode ==
  I : Inport
  Bypass diode junction temperature : Constant  Value=298
  Bypass diode saturation current : Constant  Value=3.2e-6
  Divide4 : Product  Inputs=/*
  Gain1 : Gain  Gain=Rs_bypass
  Gain2 : Gain  Gain=-1
  Gain9 : Gain  Gain=1.5
  Math Function2 : Math  Operator=log  SaturateOnIntegerOverflow=on
  Product2 : Product  RndMeth=Zero
  Saturation1 : Saturate  UpperLimit=1e24  LowerLimit=0
  Subtract : Sum
  Subtract5 : Sum
  Thermal voltage : Subsystem
  Ubypass : Outport
  wires:
  Math Function2/1 -> Product2/2
  Gain9/1 -> Product2/1
  Thermal voltage/1(Vt) -> Gain9/1
  Bypass diode saturation current/1 -> Subtract5/1, Divide4/1
  I/1 -> Saturation1/1
  Product2/1 -> Subtract/1
  Gain1/1 -> Subtract/2
  Bypass diode junction temperature/1 -> Thermal voltage/1(T)
  Divide4/1 -> Math Function2/1
  Subtract5/1 -> Divide4/2
  Saturation1/1 -> Subtract5/2, Gain1/1
  Subtract/1 -> Gain2/1
  Gain2/1 -> Ubypass/1

== system PV_string_with_MPPT/PV generator; 10 modules in series/PV module  #7/Pv module ==
  G : Inport
  T : Inport  Port=2
  I : Inport  Port=3
  Add1 : Sum  Inputs=+--
  Gain1 : Gain  Gain=Rsh
  Gain3 : Gain  Gain=(Rsh+Rs)/Rsh
  Subsystem : Subsystem
  Subsystem1 : Subsystem
  U : Outport
  Isc : Outport  Port=2
  wires:
  Subsystem/2(Ipv) -> Add1/1
  G/1 -> Subsystem/1(G)
  T/1 -> Subsystem/2(T), Subsystem1/1(T)
  Subsystem1/1(Id) -> Add1/2
  I/1 -> Subsystem1/3(I), Gain3/1
  Gain3/1 -> Add1/3
  Add1/1 -> Gain1/1
  Gain1/1 -> Subsystem1/2(U), U/1
  Subsystem/1(Isc) -> Isc/1

== system PV_string_with_MPPT/PV generator; 10 modules in series/PV module  #8/Bypass diode ==
  I : Inport
  Bypass diode junction temperature : Constant  Value=298
  Bypass diode saturation current : Constant  Value=3.2e-6
  Divide4 : Product  Inputs=/*
  Gain1 : Gain  Gain=Rs_bypass
  Gain2 : Gain  Gain=-1
  Gain9 : Gain  Gain=1.5
  Math Function2 : Math  Operator=log  SaturateOnIntegerOverflow=on
  Product2 : Product  RndMeth=Zero
  Saturation1 : Saturate  UpperLimit=1e24  LowerLimit=0
  Subtract : Sum
  Subtract5 : Sum
  Thermal voltage : Subsystem
  Ubypass : Outport
  wires:
  Gain2/1 -> Ubypass/1
  Subtract/1 -> Gain2/1
  Saturation1/1 -> Gain1/1, Subtract5/2
  Subtract5/1 -> Divide4/2
  Divide4/1 -> Math Function2/1
  Bypass diode junction temperature/1 -> Thermal voltage/1(T)
  Gain1/1 -> Subtract/2
  Product2/1 -> Subtract/1
  I/1 -> Saturation1/1
  Bypass diode saturation current/1 -> Divide4/1, Subtract5/1
  Thermal voltage/1(Vt) -> Gain9/1
  Gain9/1 -> Product2/1
  Math Function2/1 -> Product2/2

== system PV_string_with_MPPT/PV generator; 10 modules in series/PV module  #8/Pv module ==
  G : Inport
  T : Inport  Port=2
  I : Inport  Port=3
  Add1 : Sum  Inputs=+--
  Gain1 : Gain  Gain=Rsh
  Gain3 : Gain  Gain=(Rsh+Rs)/Rsh
  Subsystem : Subsystem
  Subsystem1 : Subsystem
  U : Outport
  Isc : Outport  Port=2
  wires:
  Subsystem/1(Isc) -> Isc/1
  Gain1/1 -> U/1, Subsystem1/2(U)
  Add1/1 -> Gain1/1
  Gain3/1 -> Add1/3
  I/1 -> Gain3/1, Subsystem1/3(I)
  Subsystem1/1(Id) -> Add1/2
  T/1 -> Subsystem1/1(T), Subsystem/2(T)
  G/1 -> Subsystem/1(G)
  Subsystem/2(Ipv) -> Add1/1

== system PV_string_with_MPPT/PV generator; 10 modules in series/PV module  #9/Bypass diode ==
  I : Inport
  Bypass diode junction temperature : Constant  Value=298
  Bypass diode saturation current : Constant  Value=3.2e-6
  Divide4 : Product  Inputs=/*
  Gain1 : Gain  Gain=Rs_bypass
  Gain2 : Gain  Gain=-1
  Gain9 : Gain  Gain=1.5
  Math Function2 : Math  Operator=log  SaturateOnIntegerOverflow=on
  Product2 : Product  RndMeth=Zero
  Saturation1 : Saturate  UpperLimit=1e24  LowerLimit=0
  Subtract : Sum
  Subtract5 : Sum
  Thermal voltage : Subsystem
  Ubypass : Outport
  wires:
  Math Function2/1 -> Product2/2
  Gain9/1 -> Product2/1
  Thermal voltage/1(Vt) -> Gain9/1
  Bypass diode saturation current/1 -> Subtract5/1, Divide4/1
  I/1 -> Saturation1/1
  Product2/1 -> Subtract/1
  Gain1/1 -> Subtract/2
  Bypass diode junction temperature/1 -> Thermal voltage/1(T)
  Divide4/1 -> Math Function2/1
  Subtract5/1 -> Divide4/2
  Saturation1/1 -> Subtract5/2, Gain1/1
  Subtract/1 -> Gain2/1
  Gain2/1 -> Ubypass/1

== system PV_string_with_MPPT/PV generator; 10 modules in series/PV module  #9/Pv module ==
  G : Inport
  T : Inport  Port=2
  I : Inport  Port=3
  Add1 : Sum  Inputs=+--
  Gain1 : Gain  Gain=Rsh
  Gain3 : Gain  Gain=(Rsh+Rs)/Rsh
  Subsystem : Subsystem
  Subsystem1 : Subsystem
  U : Outport
  Isc : Outport  Port=2
  wires:
  Subsystem/2(Ipv) -> Add1/1
  G/1 -> Subsystem/1(G)
  T/1 -> Subsystem/2(T), Subsystem1/1(T)
  Subsystem1/1(Id) -> Add1/2
  I/1 -> Subsystem1/3(I), Gain3/1
  Gain3/1 -> Add1/3
  Add1/1 -> Gain1/1
  Gain1/1 -> Subsystem1/2(U), U/1
  Subsystem/1(Isc) -> Isc/1

== system PV_string_with_MPPT/PV generator; 10 modules in series/PV module  #1/Bypass diode/Thermal voltage ==
  T : Inport
  Constant5 : Constant  Value=k/q
  Product : Product  RndMeth=Zero
  Vt : Outport
  wires:
  Product/1 -> Vt/1
  T/1 -> Product/1
  Constant5/1 -> Product/2

== system PV_string_with_MPPT/PV generator; 10 modules in series/PV module  #1/Pv module/Subsystem ==
  G : Inport
  T : Inport  Port=2
  Add : Sum
  Constant : Constant  Value=Isc_stc
  Constant1 : Constant  Value=T_stc
  Constant2 : Constant  Value=G_stc
  Divide : Product  Inputs=*/
  Gain : Gain  Gain=Ki
  Gain1 : Gain  Gain=(Rsh+Rs)/Rsh
  Product1 : Product  RndMeth=Zero
  Subtract : Sum  Inputs=+-
  Isc : Outport
  Ipv : Outport  Port=2
  wires:
  Gain1/1 -> Ipv/1
  Product1/1 -> Isc/1, Gain1/1
  Divide/1 -> Product1/2
  Add/1 -> Product1/1
  G/1 -> Divide/1
  T/1 -> Subtract/1
  Constant2/1 -> Divide/2
  Subtract/1 -> Gain/1
  Constant1/1 -> Subtract/2
  Gain/1 -> Add/2
  Constant/1 -> Add/1

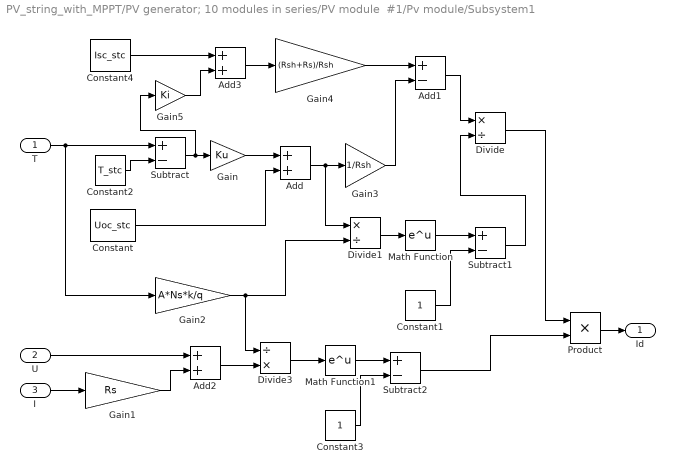
== system PV_string_with_MPPT/PV generator; 10 modules in series/PV module  #1/Pv module/Subsystem1 ==
  T : Inport
  U : Inport  Port=2
  I : Inport  Port=3
  Add : Sum
  Add1 : Sum  Inputs=+-
  Add2 : Sum
  Add3 : Sum
  Constant : Constant  Value=Uoc_stc
  Constant1 : Constant
  Constant2 : Constant  Value=T_stc
  Constant3 : Constant
  Constant4 : Constant  Value=Isc_stc
  Divide : Product  Inputs=*/
  Divide1 : Product  Inputs=*/
  Divide3 : Product  Inputs=/*
  Gain : Gain  Gain=Ku
  Gain1 : Gain  Gain=Rs
  Gain2 : Gain  Gain=A*Ns*k/q
  Gain3 : Gain  Gain=1/Rsh
  Gain4 : Gain  Gain=(Rsh+Rs)/Rsh
  Gain5 : Gain  Gain=Ki
  Math Function : Math  SaturateOnIntegerOverflow=on
  Math Function1 : Math  SaturateOnIntegerOverflow=on
  Product : Product  RndMeth=Zero
  Subtract : Sum  Inputs=+-
  Subtract1 : Sum  Inputs=+-
  Subtract2 : Sum  Inputs=+-
  Id : Outport
  wires:
  Gain4/1 -> Add1/1
  Subtract/1 -> Gain5/1, Gain/1
  Constant/1 -> Add/2
  Gain/1 -> Add/1
  Add3/1 -> Gain4/1
  Gain5/1 -> Add3/2
  Gain3/1 -> Add1/2
  Gain1/1 -> Add2/2
  I/1 -> Gain1/1
  Add/1 -> Gain3/1, Divide1/1
  Product/1 -> Id/1
  Subtract2/1 -> Product/2
  Constant3/1 -> Subtract2/2
  Math Function1/1 -> Subtract2/1
  Divide3/1 -> Math Function1/1
  Add2/1 -> Divide3/2
  U/1 -> Add2/1
  Divide/1 -> Product/1
  Subtract1/1 -> Divide/2
  Math Function/1 -> Subtract1/1
  Divide1/1 -> Math Function/1
  Gain2/1 -> Divide3/1, Divide1/2
  Constant1/1 -> Subtract1/2
  Add1/1 -> Divide/1
  T/1 -> Gain2/1, Subtract/1
  Constant2/1 -> Subtract/2
  Constant4/1 -> Add3/1

== system PV_string_with_MPPT/PV generator; 10 modules in series/PV module  #10/Bypass diode/Thermal voltage ==
  T : Inport
  Constant5 : Constant  Value=k/q
  Product : Product  RndMeth=Zero
  Vt : Outport
  wires:
  Product/1 -> Vt/1
  T/1 -> Product/1
  Constant5/1 -> Product/2

== system PV_string_with_MPPT/PV generator; 10 modules in series/PV module  #10/Pv module/Subsystem ==
  G : Inport
  T : Inport  Port=2
  Add : Sum
  Constant : Constant  Value=Isc_stc
  Constant1 : Constant  Value=T_stc
  Constant2 : Constant  Value=G_stc
  Divide : Product  Inputs=*/
  Gain : Gain  Gain=Ki
  Gain1 : Gain  Gain=(Rsh+Rs)/Rsh
  Product1 : Product  RndMeth=Zero
  Subtract : Sum  Inputs=+-
  Isc : Outport
  Ipv : Outport  Port=2
  wires:
  Gain1/1 -> Ipv/1
  Product1/1 -> Isc/1, Gain1/1
  Divide/1 -> Product1/2
  Add/1 -> Product1/1
  G/1 -> Divide/1
  T/1 -> Subtract/1
  Constant2/1 -> Divide/2
  Subtract/1 -> Gain/1
  Constant1/1 -> Subtract/2
  Gain/1 -> Add/2
  Constant/1 -> Add/1

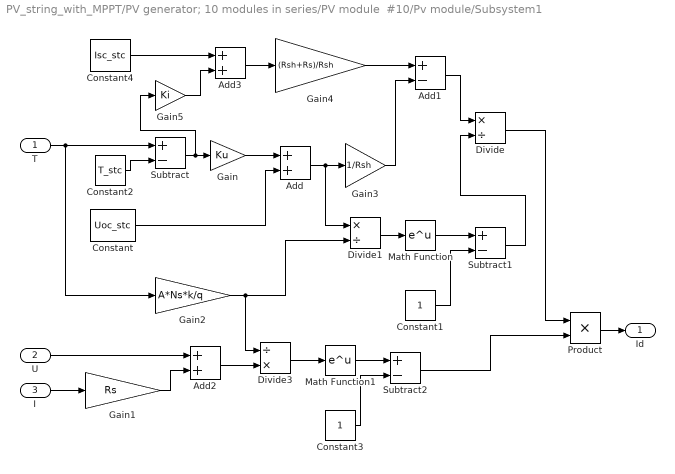
== system PV_string_with_MPPT/PV generator; 10 modules in series/PV module  #10/Pv module/Subsystem1 ==
  T : Inport
  U : Inport  Port=2
  I : Inport  Port=3
  Add : Sum
  Add1 : Sum  Inputs=+-
  Add2 : Sum
  Add3 : Sum
  Constant : Constant  Value=Uoc_stc
  Constant1 : Constant
  Constant2 : Constant  Value=T_stc
  Constant3 : Constant
  Constant4 : Constant  Value=Isc_stc
  Divide : Product  Inputs=*/
  Divide1 : Product  Inputs=*/
  Divide3 : Product  Inputs=/*
  Gain : Gain  Gain=Ku
  Gain1 : Gain  Gain=Rs
  Gain2 : Gain  Gain=A*Ns*k/q
  Gain3 : Gain  Gain=1/Rsh
  Gain4 : Gain  Gain=(Rsh+Rs)/Rsh
  Gain5 : Gain  Gain=Ki
  Math Function : Math  SaturateOnIntegerOverflow=on
  Math Function1 : Math  SaturateOnIntegerOverflow=on
  Product : Product  RndMeth=Zero
  Subtract : Sum  Inputs=+-
  Subtract1 : Sum  Inputs=+-
  Subtract2 : Sum  Inputs=+-
  Id : Outport
  wires:
  Gain4/1 -> Add1/1
  Subtract/1 -> Gain5/1, Gain/1
  Constant/1 -> Add/2
  Gain/1 -> Add/1
  Add3/1 -> Gain4/1
  Gain5/1 -> Add3/2
  Gain3/1 -> Add1/2
  Gain1/1 -> Add2/2
  I/1 -> Gain1/1
  Add/1 -> Gain3/1, Divide1/1
  Product/1 -> Id/1
  Subtract2/1 -> Product/2
  Constant3/1 -> Subtract2/2
  Math Function1/1 -> Subtract2/1
  Divide3/1 -> Math Function1/1
  Add2/1 -> Divide3/2
  U/1 -> Add2/1
  Divide/1 -> Product/1
  Subtract1/1 -> Divide/2
  Math Function/1 -> Subtract1/1
  Divide1/1 -> Math Function/1
  Gain2/1 -> Divide3/1, Divide1/2
  Constant1/1 -> Subtract1/2
  Add1/1 -> Divide/1
  T/1 -> Gain2/1, Subtract/1
  Constant2/1 -> Subtract/2
  Constant4/1 -> Add3/1

== system PV_string_with_MPPT/PV generator; 10 modules in series/PV module  #2/Bypass diode/Thermal voltage ==
  T : Inport
  Constant5 : Constant  Value=k/q
  Product : Product  RndMeth=Zero
  Vt : Outport
  wires:
  Constant5/1 -> Product/2
  T/1 -> Product/1
  Product/1 -> Vt/1

== system PV_string_with_MPPT/PV generator; 10 modules in series/PV module  #2/Pv module/Subsystem ==
  G : Inport
  T : Inport  Port=2
  Add : Sum
  Constant : Constant  Value=Isc_stc
  Constant1 : Constant  Value=T_stc
  Constant2 : Constant  Value=G_stc
  Divide : Product  Inputs=*/
  Gain : Gain  Gain=Ki
  Gain1 : Gain  Gain=(Rsh+Rs)/Rsh
  Product1 : Product  RndMeth=Zero
  Subtract : Sum  Inputs=+-
  Isc : Outport
  Ipv : Outport  Port=2
  wires:
  Constant/1 -> Add/1
  Gain/1 -> Add/2
  Constant1/1 -> Subtract/2
  Subtract/1 -> Gain/1
  Constant2/1 -> Divide/2
  T/1 -> Subtract/1
  G/1 -> Divide/1
  Add/1 -> Product1/1
  Divide/1 -> Product1/2
  Product1/1 -> Gain1/1, Isc/1
  Gain1/1 -> Ipv/1

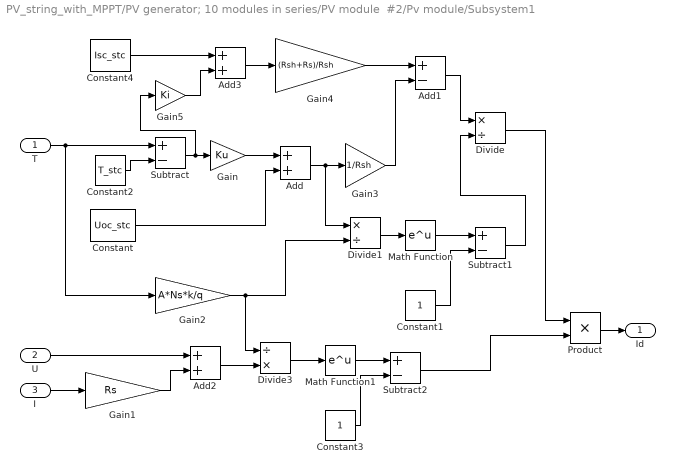
== system PV_string_with_MPPT/PV generator; 10 modules in series/PV module  #2/Pv module/Subsystem1 ==
  T : Inport
  U : Inport  Port=2
  I : Inport  Port=3
  Add : Sum
  Add1 : Sum  Inputs=+-
  Add2 : Sum
  Add3 : Sum
  Constant : Constant  Value=Uoc_stc
  Constant1 : Constant
  Constant2 : Constant  Value=T_stc
  Constant3 : Constant
  Constant4 : Constant  Value=Isc_stc
  Divide : Product  Inputs=*/
  Divide1 : Product  Inputs=*/
  Divide3 : Product  Inputs=/*
  Gain : Gain  Gain=Ku
  Gain1 : Gain  Gain=Rs
  Gain2 : Gain  Gain=A*Ns*k/q
  Gain3 : Gain  Gain=1/Rsh
  Gain4 : Gain  Gain=(Rsh+Rs)/Rsh
  Gain5 : Gain  Gain=Ki
  Math Function : Math  SaturateOnIntegerOverflow=on
  Math Function1 : Math  SaturateOnIntegerOverflow=on
  Product : Product  RndMeth=Zero
  Subtract : Sum  Inputs=+-
  Subtract1 : Sum  Inputs=+-
  Subtract2 : Sum  Inputs=+-
  Id : Outport
  wires:
  Constant4/1 -> Add3/1
  Constant2/1 -> Subtract/2
  T/1 -> Subtract/1, Gain2/1
  Add1/1 -> Divide/1
  Constant1/1 -> Subtract1/2
  Gain2/1 -> Divide1/2, Divide3/1
  Divide1/1 -> Math Function/1
  Math Function/1 -> Subtract1/1
  Subtract1/1 -> Divide/2
  Divide/1 -> Product/1
  U/1 -> Add2/1
  Add2/1 -> Divide3/2
  Divide3/1 -> Math Function1/1
  Math Function1/1 -> Subtract2/1
  Constant3/1 -> Subtract2/2
  Subtract2/1 -> Product/2
  Product/1 -> Id/1
  Add/1 -> Divide1/1, Gain3/1
  I/1 -> Gain1/1
  Gain1/1 -> Add2/2
  Gain3/1 -> Add1/2
  Gain5/1 -> Add3/2
  Add3/1 -> Gain4/1
  Gain/1 -> Add/1
  Constant/1 -> Add/2
  Subtract/1 -> Gain/1, Gain5/1
  Gain4/1 -> Add1/1

== system PV_string_with_MPPT/PV generator; 10 modules in series/PV module  #3/Bypass diode/Thermal voltage ==
  T : Inport
  Constant5 : Constant  Value=k/q
  Product : Product  RndMeth=Zero
  Vt : Outport
  wires:
  Product/1 -> Vt/1
  T/1 -> Product/1
  Constant5/1 -> Product/2

== system PV_string_with_MPPT/PV generator; 10 modules in series/PV module  #3/Pv module/Subsystem ==
  G : Inport
  T : Inport  Port=2
  Add : Sum
  Constant : Constant  Value=Isc_stc
  Constant1 : Constant  Value=T_stc
  Constant2 : Constant  Value=G_stc
  Divide : Product  Inputs=*/
  Gain : Gain  Gain=Ki
  Gain1 : Gain  Gain=(Rsh+Rs)/Rsh
  Product1 : Product  RndMeth=Zero
  Subtract : Sum  Inputs=+-
  Isc : Outport
  Ipv : Outport  Port=2
  wires:
  Gain1/1 -> Ipv/1
  Product1/1 -> Isc/1, Gain1/1
  Divide/1 -> Product1/2
  Add/1 -> Product1/1
  G/1 -> Divide/1
  T/1 -> Subtract/1
  Constant2/1 -> Divide/2
  Subtract/1 -> Gain/1
  Constant1/1 -> Subtract/2
  Gain/1 -> Add/2
  Constant/1 -> Add/1

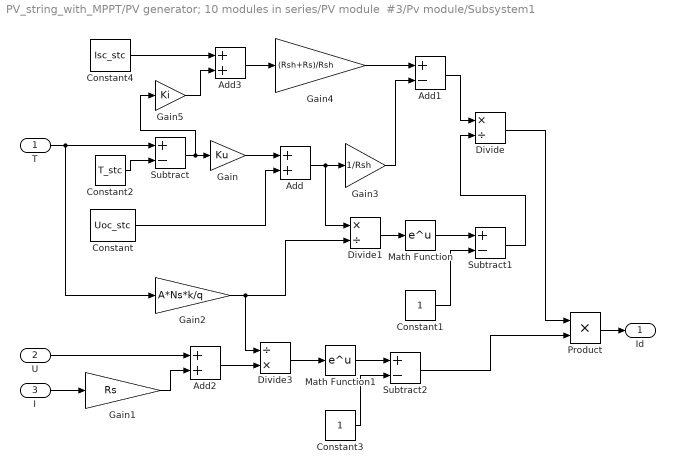
== system PV_string_with_MPPT/PV generator; 10 modules in series/PV module  #3/Pv module/Subsystem1 ==
  T : Inport
  U : Inport  Port=2
  I : Inport  Port=3
  Add : Sum
  Add1 : Sum  Inputs=+-
  Add2 : Sum
  Add3 : Sum
  Constant : Constant  Value=Uoc_stc
  Constant1 : Constant
  Constant2 : Constant  Value=T_stc
  Constant3 : Constant
  Constant4 : Constant  Value=Isc_stc
  Divide : Product  Inputs=*/
  Divide1 : Product  Inputs=*/
  Divide3 : Product  Inputs=/*
  Gain : Gain  Gain=Ku
  Gain1 : Gain  Gain=Rs
  Gain2 : Gain  Gain=A*Ns*k/q
  Gain3 : Gain  Gain=1/Rsh
  Gain4 : Gain  Gain=(Rsh+Rs)/Rsh
  Gain5 : Gain  Gain=Ki
  Math Function : Math  SaturateOnIntegerOverflow=on
  Math Function1 : Math  SaturateOnIntegerOverflow=on
  Product : Product  RndMeth=Zero
  Subtract : Sum  Inputs=+-
  Subtract1 : Sum  Inputs=+-
  Subtract2 : Sum  Inputs=+-
  Id : Outport
  wires:
  Gain4/1 -> Add1/1
  Subtract/1 -> Gain5/1, Gain/1
  Constant/1 -> Add/2
  Gain/1 -> Add/1
  Add3/1 -> Gain4/1
  Gain5/1 -> Add3/2
  Gain3/1 -> Add1/2
  Gain1/1 -> Add2/2
  I/1 -> Gain1/1
  Add/1 -> Gain3/1, Divide1/1
  Product/1 -> Id/1
  Subtract2/1 -> Product/2
  Constant3/1 -> Subtract2/2
  Math Function1/1 -> Subtract2/1
  Divide3/1 -> Math Function1/1
  Add2/1 -> Divide3/2
  U/1 -> Add2/1
  Divide/1 -> Product/1
  Subtract1/1 -> Divide/2
  Math Function/1 -> Subtract1/1
  Divide1/1 -> Math Function/1
  Gain2/1 -> Divide3/1, Divide1/2
  Constant1/1 -> Subtract1/2
  Add1/1 -> Divide/1
  T/1 -> Gain2/1, Subtract/1
  Constant2/1 -> Subtract/2
  Constant4/1 -> Add3/1

== system PV_string_with_MPPT/PV generator; 10 modules in series/PV module  #4/Bypass diode/Thermal voltage ==
  T : Inport
  Constant5 : Constant  Value=k/q
  Product : Product  RndMeth=Zero
  Vt : Outport
  wires:
  Constant5/1 -> Product/2
  T/1 -> Product/1
  Product/1 -> Vt/1

== system PV_string_with_MPPT/PV generator; 10 modules in series/PV module  #4/Pv module/Subsystem ==
  G : Inport
  T : Inport  Port=2
  Add : Sum
  Constant : Constant  Value=Isc_stc
  Constant1 : Constant  Value=T_stc
  Constant2 : Constant  Value=G_stc
  Divide : Product  Inputs=*/
  Gain : Gain  Gain=Ki
  Gain1 : Gain  Gain=(Rsh+Rs)/Rsh
  Product1 : Product  RndMeth=Zero
  Subtract : Sum  Inputs=+-
  Isc : Outport
  Ipv : Outport  Port=2
  wires:
  Constant/1 -> Add/1
  Gain/1 -> Add/2
  Constant1/1 -> Subtract/2
  Subtract/1 -> Gain/1
  Constant2/1 -> Divide/2
  T/1 -> Subtract/1
  G/1 -> Divide/1
  Add/1 -> Product1/1
  Divide/1 -> Product1/2
  Product1/1 -> Gain1/1, Isc/1
  Gain1/1 -> Ipv/1
